simulink model "Mainframe"  (R2021a)
settings: Solver=FixedStepAuto  StartTime=0.0  StopTime=60  FixedStep=0.001  RelTol=1e-3
values from neighbouring files (symbols this model uses):
  den_lpf_d = den_lpf20    [Mainframe_init.m]    (also in load_autopilot.m)
  Emulated_FCC_IO_Delay = 7    [Mainframe_init.m]
  Enable_Gyros = 0    [Mainframe_init.m]
  Enable_INS = 0    [Mainframe_init.m]
  num_lpf_d = num_lpf20    [Mainframe_init.m]    (also in load_autopilot.m)
undefined symbols (not defined in the file or in its folder): act_dmp, act_omega, Actuator, Aerodynamics, aMode, Autopilot, AUX, c_b_WGS, c_be, c_flat, c_grav, c_h_geop0, c_h_geope, c_pa0, c_pe, c_r0, c_rot, c_rsma, c_Tmp0, d_siB_0, d_siB_max, d_siB_min, dd_siB_max, dd_siB_min, dev, DiscIntNeverNeededParam, e_pa, e_Tmp, fin_maxrate, flag_I_act_switch, flag_I_aero_switch, flag_I_flat, flag_I_gravity_switch, flag_I_rot, hcr, HIL_Data, JMMM_0, JMMM_e, JSPB_e, lat_0, lon_0, Mass_Props, mB_0, mM_0, mM_e, National_Instruments, Newton, pBII_0, PCIe, pMPB, pNPB, propellant_kg, prp_FBPB, prp_mdot, prp_T, pSPB, pwm_output1, qEG_0, qIB_0, qIE_0 ... (+31)
libraries: simulink_extras x38, simulink x31, custom_blocks x11, sldrtlib x10, aerolibcommonsys x4, px4Sensorslib x3, px4lib x3, aerolibnav x1
(part 2 of 17)

== system Mainframe/Non-linear Flight Dynamic Model/GRM_Airframe ==
  siB_cmd : Inport
  T_sim_glbl : Inport  Port=2
  Bus Creator : BusCreator  Inputs=9
  aerodynamics : Subsystem
  environment : Subsystem
  fin_actuators : Subsystem
  forces_moments : Subsystem
  gravity : Subsystem
  input : Subsystem
  motion_kinematics : Subsystem
  propulsion : Subsystem
  rb_eom : Subsystem
  stream_flow : Subsystem
  weight_and_balance : Subsystem
  airfr : Outport  VectorParamsAs1DForOutWhenUnconnected=off
  wires:
  forces_moments/1(for_mom_bus) -> rb_eom/2(for_mom)
  [env] -> Bus Creator/9
  [fin] -> Bus Creator/7
  [motion_kin] -> Bus Creator/6
  [env_glbl] -> aerodynamics/4(env_glbl)
  aerodynamics/1(aero) -> forces_moments/1(aero), [aero]
  [motion_kin] -> rb_eom/1(mot_kin)
  weight_and_balance/1(wab) -> rb_eom/3(wab), gravity/2(wab), [wab], propulsion/2(wab)
  [wab] -> aerodynamics/3(wab)
  [str_flow] -> Bus Creator/5
  [motion_kin] -> forces_moments/2(motion_kin)
  motion_kinematics/1(motion_kin) -> stream_flow/2(motion_kin), [motion_kin]
  [grav] -> Bus Creator/3
  Bus Creator/1 -> airfr/1  "airfr_bus"
  [aero] -> Bus Creator/4
  environment/1(env) -> [env], stream_flow/3(env), gravity/1(env)
  [prp] -> forces_moments/4(prp)
  [prp] -> Bus Creator/8
  stream_flow/1(str_flow) -> [str_flow], aerodynamics/1(str_flow)
  input/1(cmd_bus) -> fin_actuators/1(cmd)
  [wab] -> Bus Creator/2
  gravity/1(grav) -> [grav], forces_moments/3(grav)
  T_sim_glbl/1 -> [env_glbl], environment/2(env_glbl), weight_and_balance/1(env_glb), propulsion/1(env_glbl)
  siB_cmd/1 -> input/1(siB_cmd)
  rb_eom/1(flight_dyn) -> environment/1(flight_dyn), motion_kinematics/1(flight_dyn), stream_flow/1(flight_dyn), Bus Creator/1
  fin_actuators/1(fin) -> [fin], aerodynamics/2(fin)
  propulsion/1(prp) -> [prp]

== system Mainframe/Non-linear Flight Dynamic Model/Stop-Condition ==
  States : Inport
  AND : Logic  Inputs=3  IconShape=distinctive  AllPortsSameDT=off  OutDataTypeStr=boolean
  Bus Selector1 : BusSelector  OutputSignals=POS_NED.POS_z_NED_m,POS_NED_dot.POS_z_NED_dot_m
  Compare To Constant : Subsystem  mask(Compare To Constant){relop=>, const=-700, OutDataTypeStr=boolean, ZeroCross=on}
      mask prompts: relop "Simulink:masks:Operator_MP"; const "Simulink:masks:ConstantValue_MP"; OutDataTypeStr "Simulink:masks:OutputDataType_MP"; ZeroCross "Simulink:masks:EnableZerocrossingDetection_MP"
      mask help: Simulink:masks:CompareToConstant_MD
      mask init:
      | blkName = gcb;
      | 
      | if strcmp(get_param(gcbh,'OutDataTypeStr'),'boolean')
      | 	setValue = 'boolean';
      | else
      | 	setValue = 'fixdt(0, 8)';
      | end
      | 
      | set_param([blkName,'/Compare'],'relop',relop, ...
      | 	'OutDataTypeStr', setValue, 'ZeroCross', ZeroCross);
      | 
      | str = [relop,' C']; %default
      | 
      | const_str = get_param(blkName, 'const');
      | const_val = str2num(const_str);
      | 
      | if isempty(const_val) %#ok<ST2NM>
      |     %Expression/Variable
      |     str = [relop, ' ', strtrim(const_str)];
      | else
      |     if length(const_val) == 1 
      |         if Simulink.data.isSupportedEnumClass(class(const_val))
      |             % Special Handling for Enumerations
      |             if Simulink.data.getEnumTypeInfo(class(const_val), 'AddClassNameToEnumNames')
      |                 str = [relop, ' ', strtrim(const_str)];
      |             else
      |                 str = [relop, ' ', char(const_val)];
      |             end
      |         elseif(isfloat(const_val) || isinteger(const_val) || islogical(const_val)) 
      |                 str = [relop, ' ', num2str(const_val)];
      |         end
      |     end
      | end
      mask TypeOptions relop: == | ~= | < | <= | >= | >
      mask TypeOptions OutDataTypeStr: Simulink:masks:uint8 | Simulink:masks:boolean
      mask Callback ZeroCross: sl('zeroCrossEnable', gcbh);
      mask Display: disp(str)
  Compare To Constant1 : Subsystem  mask(Compare To Constant){relop=>, const=0, OutDataTypeStr=boolean, ZeroCross=on}
      mask prompts: relop "Simulink:masks:Operator_MP"; const "Simulink:masks:ConstantValue_MP"; OutDataTypeStr "Simulink:masks:OutputDataType_MP"; ZeroCross "Simulink:masks:EnableZerocrossingDetection_MP"
      mask help: Simulink:masks:CompareToConstant_MD
      mask init: same as Mainframe/Non-linear Flight Dynamic Model/Stop-Condition/Compare To Constant
      mask TypeOptions relop: == | ~= | < | <= | >= | >
      mask TypeOptions OutDataTypeStr: Simulink:masks:uint8 | Simulink:masks:boolean
      mask Callback ZeroCross: sl('zeroCrossEnable', gcbh);
      mask Display: disp(str)
  From4 : From  Commented=on  GotoTag=HIL_Ready  TagVisibility=global
  Stop Simulation : Stop
  wires:
  Bus Selector1/1 -> Compare To Constant/1(u)  "<POS_z_NED_m>"
  States/1 -> Bus Selector1/1
  Compare To Constant/1(y) -> AND/2
  AND/1 -> Stop Simulation/1
  From4/1 -> AND/1
  Bus Selector1/2 -> Compare To Constant1/1(u)  "<POS_z_NED_dot_m>"
  Compare To Constant1/1(y) -> AND/3

== system Mainframe/Non-linear Flight Dynamic Model/Subsystem1 ==
  Control Surface Deflections : Inport
  Envoronment : Inport  Port=2
  Enable : EnablePort
  Extract States : Subsystem
  Fin Deflections : Subsystem
  GRM_Airframe : Subsystem
      mask Display: image('$imagefile'); % Use "Edit Image" on toolstrip to change.
  Missile States : Outport
  wires:
  GRM_Airframe/1(airfr) -> Extract States/1(airfr_bus)
  Control Surface Deflections/1 -> Fin Deflections/1(Servo Deflections)
  Envoronment/1 -> GRM_Airframe/2(T_sim_glbl)
  Extract States/1(States) -> Missile States/1
  Fin Deflections/1(afinB) -> GRM_Airframe/1(siB_cmd)

== system Mainframe/Non-linear Flight Dynamic Model/Translate Fins ==
  Servo Deflections : Inport
  Add : Sum
  Bus Selector : BusSelector  OutputSignals=Fin_1,Fin_2,Fin_3,Fin_4
  Constant1 : Constant  Value=unc_fin_def_roll
  Constant2 : Constant  Value=unc_fin_def_pitch
  Constant3 : Constant  Value=unc_fin_def_yaw
  Degrees to Radians : Subsystem  mask(DegreesToRadians){}
      mask help: SimulinkBlocks:simulink_extras:DegreesToRadians_MD
      mask Help: web([docroot '/simulink/ref_extras/degreestoradians.html'])
      mask Display: disp('D2R')
  Degrees to Radians1 : Subsystem  mask(DegreesToRadians){}
      mask help: SimulinkBlocks:simulink_extras:DegreesToRadians_MD
      mask Help: web([docroot '/simulink/ref_extras/degreestoradians.html'])
      mask Display: disp('D2R')
  Degrees to Radians2 : Subsystem  mask(DegreesToRadians){}
      mask help: SimulinkBlocks:simulink_extras:DegreesToRadians_MD
      mask Help: web([docroot '/simulink/ref_extras/degreestoradians.html'])
      mask Display: disp('D2R')
  Vector Concatenate : Concatenate  NumInputs=4
  Vector Concatenate1 : Concatenate  NumInputs=3
  control_allocation : Subsystem
  afinB : Outport
  wires:
  Degrees to Radians2/1(Radians out) -> Vector Concatenate1/3
  Vector Concatenate1/1 -> control_allocation/1(fin_cmd)  "fin_cmd"
  Constant1/1 -> Degrees to Radians/1(Degrees in)  "xi_cmd"
  Degrees to Radians1/1(Radians out) -> Vector Concatenate1/2
  Degrees to Radians/1(Radians out) -> Vector Concatenate1/1
  Constant3/1 -> Degrees to Radians2/1(Degrees in)  "ze_cmd"
  Constant2/1 -> Degrees to Radians1/1(Degrees in)  "et_cmd"
  Bus Selector/2 -> Vector Concatenate/2  "<Fin_2>"
  Servo Deflections/1 -> Bus Selector/1
  Bus Selector/1 -> Vector Concatenate/1  "<Fin_1>"
  Bus Selector/4 -> Vector Concatenate/4  "<Fin_4>"
  Vector Concatenate/1 -> Add/1
  Bus Selector/3 -> Vector Concatenate/3  "<Fin_3>"
  control_allocation/1(siB_cmd) -> Add/2
  Add/1 -> afinB/1  "siB_cmd"

== system Mainframe/Real FCC/Enabled Subsystem ==
  Hold : Inport
  Trigger : TriggerPort  VariantControl=Variant  PortDimensions=1
  Pass : Outport
  wires:
  Hold/1 -> Pass/1

== system Mainframe/Real Servos/Reset Encoders ==
  Reset Encoders : Inport
  Encoder Readings : Inport  Port=2
  NOT : Logic  Operator=NOT  IconShape=distinctive  AllPortsSameDT=off  OutDataTypeStr=boolean
  Sum : Sum  Inputs=-+|
  Triggered Subsystem : Subsystem  TreatAsAtomicUnit=on
  Fin Angles : Outport
  wires:
  Encoder Readings/1 -> Sum/2, Triggered Subsystem/1(In1)
  Triggered Subsystem/1(Out1) -> Sum/1
  Reset Encoders/1 -> NOT/1
  Sum/1 -> Fin Angles/1
  NOT/1 -> Triggered Subsystem/Enable

== system Mainframe/Servos/Emulated Servos ==
  FCC Data : Inport
  Bus Creator : BusCreator  Inputs=4
  Bus Selector : BusSelector  OutputSignals=Control Surface Cmd.Fin_1_Cmd_rad,Control Surface Cmd.Fin_2_Cmd_rad,Control Surface Cmd.Fin_3_Cmd_rad,Control Surface Cmd.Fin_4_Cmd_rad
  Transfer Fcn{1..4} (4 alike) : TransferFcn  Numerator=33770  Denominator=[1 395.7 33770]
  Fin Deflections : Outport
  wires:
  FCC Data/1 -> Bus Selector/1
  Bus Selector/1 -> Transfer Fcn1/1  "<Fin_1_Cmd_rad>"
  Bus Selector/2 -> Transfer Fcn2/1  "<Fin_2_Cmd_rad>"
  Bus Selector/3 -> Transfer Fcn3/1  "<Fin_3_Cmd_rad>"
  Bus Selector/4 -> Transfer Fcn4/1  "<Fin_4_Cmd_rad>"
  Bus Creator/1 -> Fin Deflections/1
  Transfer Fcn1/1 -> Bus Creator/1  "Fin_1"
  Transfer Fcn2/1 -> Bus Creator/2  "Fin_2"
  Transfer Fcn3/1 -> Bus Creator/3  "Fin_3"
  Transfer Fcn4/1 -> Bus Creator/4  "Fin_4"

== system Mainframe/Servos/Real Servos ==
  FCC Data : Inport
  Bus Creator : BusCreator  Inputs=4
  Demux : Demux
  Encoder Input : sldrtlib/Encoder Input  SampleTime=0.001  MaxMissedTicks=10  ShowMissedTicks=off  YieldWhenWaiting=off  DrvName=National_Instruments/PCIe-6321  DrvAddress=4294967295  DrvOptions=[0 0 0 2 2 2 2]  Channels=1:4  QuadMode=3  IndexPulse=1  InputFilter=Inf  DataType=1
      settings: AttributesFormatString=National Instruments\nPCIe-6321 [auto]
  Reset Encoders : Subsystem
  Terminator : Terminator
  Ticks to rads : Gain  Gain=2*pi/4096
  Fin Deflections : Outport
  wires:
  Encoder Input/1 -> Ticks to rads/1
  FCC Data/1 -> Terminator/1
  Bus Creator/1 -> Fin Deflections/1
  Demux/3 -> Bus Creator/3  "Fin_3"
  Demux/2 -> Bus Creator/2  "Fin_2"
  Demux/1 -> Bus Creator/1  "Fin_1"
  Demux/4 -> Bus Creator/4  "Fin_4"
  [HIL_Ready] -> Reset Encoders/1(Reset Encoders)
  Ticks to rads/1 -> Reset Encoders/2(Encoder Readings)
  Reset Encoders/1(Fin Angles) -> Demux/1

== system Mainframe/Virtual IMU/Gravity Vector ==
  Phi : Inport
  Theta : Inport  Port=2
  Cos : Trigonometry
  Cos1 : Trigonometry
  Cos2 : Trigonometry  Operator=cos
  Cos3 : Trigonometry  Operator=cos
  Multiply : Gain  Gain=9.81
  Multiply1 : Gain  Gain=9.81
  Multiply2 : Gain  Gain=-9.81
  Product : Product
  Product1 : Product
  Vector Concatenate1 : Concatenate  NumInputs=3
  g : Outport
  wires:
  Vector Concatenate1/1 -> g/1
  Cos/1 -> Multiply2/1
  Product/1 -> Multiply/1
  Cos1/1 -> Product/1
  Theta/1 -> Cos/1, Cos2/1
  Multiply/1 -> Vector Concatenate1/2
  Phi/1 -> Cos3/1, Cos1/1
  Product1/1 -> Multiply1/1
  Multiply1/1 -> Vector Concatenate1/3
  Multiply2/1 -> Vector Concatenate1/1
  Cos2/1 -> Product1/1, Product/2
  Cos3/1 -> Product1/2

== system Mainframe/Emulated FCC/Emulated Pixhawk/Autopilot ==
  Cmd : Inport
  IMU Data : Inport  Port=2
  INS Data : Inport  Port=3
  Bus Creator3 : BusCreator  Inputs=3
  Bus Selector : BusSelector  OutputSignals=phi_cmd
  Bus Selector1 : BusSelector  OutputSignals=gyro_x
  Bus Selector2 : BusSelector  OutputSignals=phi,z,p
  Calculate U : Subsystem
  Discrete Transfer Fcn : DiscreteTransferFcn  Numerator=[num_lpf_d]  Denominator=[den_lpf_d]
  Gain : Gain  Gain=-1
  Manual Switch : ManualSwitch
  Phi_Control : Subsystem
  Zero : Constant  Value=0  OutDataTypeStr=Inherit: Inherit via back propagation
  Attitude_Commands : Outport  VectorParamsAs1DForOutWhenUnconnected=off
  wires:
  Bus Selector1/1 -> Discrete Transfer Fcn/1  "<gyro_x>"
  IMU Data/1 -> Bus Selector1/1
  Calculate U/1(U) -> Phi_Control/5(V_mps)
  Zero/1 -> [Delta_Cmd_Psi], [Delta_Cmd_Theta]
  [Delta_Cmd_Phi] -> Bus Creator3/1  "Phi_Cmd_rad"
  [Delta_Cmd_Theta] -> Bus Creator3/2  "Theta_Cmd_rad"
  Bus Creator3/1 -> Attitude_Commands/1
  [Delta_Cmd_Psi] -> Bus Creator3/3  "Psi_Cmd_rad"
  Bus Selector/1 -> Phi_Control/1(phi_cmd_rad)  "<phi_cmd>"
  Cmd/1 -> Bus Selector/1
  INS Data/1 -> Calculate U/1(INS Data), Bus Selector2/1
  Bus Selector2/1 -> Phi_Control/2(phi_rad)  "<phi>"
  [rst] -> Phi_Control/4(Reset Integrators)
  Bus Selector2/2 -> Gain/1  "<z>"
  Gain/1 -> Phi_Control/6(h_m)
  Phi_Control/1(dela_cmd_rad) -> [Delta_Cmd_Phi]  "Phi_Cmd_rad"
  Discrete Transfer Fcn/1 -> Manual Switch/1
  Bus Selector2/3 -> Manual Switch/2  "<p>"
  Manual Switch/1 -> Phi_Control/3(p_rps)

== system Mainframe/Emulated FCC/Emulated Pixhawk/Convert to Bus ==
  Input : Inport  OutDataTypeStr=single
  100Hz Reset : Subsystem
  Bus Creator1 : BusCreator  Inputs=6
  Bus Creator2 : BusCreator  Inputs=12
  Bus Creator3 : BusCreator  Inputs=1
  Demux : Demux  Outputs=23
  Heartbeat : Outport  InitialOutput=0
  Ext. Commands : Outport  Port=2  OutDataTypeStr=single  InitialOutput=0
  Enable INS Flag : Outport  Port=3  InitialOutput=0
  Missile States : Outport  Port=4  OutDataTypeStr=single  InitialOutput=[0 0 0 0 0 0 0 0 0 0]
  Real Gyros Flag : Outport  Port=5  InitialOutput=0
  Virtual IMU Data : Outport  Port=6  OutDataTypeStr=single  InitialOutput=[0 0 0 0 0 0 0 0 0 0]
  tag scope: FCC_Enable=global, rst=global
  wires:
  Demux/22 -> Bus Creator2/12  "psi"
  Demux/21 -> Bus Creator2/11  "theta"
  Demux/20 -> Bus Creator2/10  "phi"
  Demux/4 -> Real Gyros Flag/1  "Real Gyros Flag"
  Demux/5 -> Bus Creator2/1  "u"
  Demux/18 -> Bus Creator1/5  "gyro_y"
  Bus Creator1/1 -> Virtual IMU Data/1
  Demux/16 -> Bus Creator1/3  "acc_z"
  Demux/9 -> Bus Creator2/5  "y"
  Demux/14 -> Bus Creator1/1  "acc_x"
  Demux/17 -> Bus Creator1/4  "gyro_x"
  Demux/15 -> Bus Creator1/2  "acc_y"
  Demux/19 -> Bus Creator1/6  "gyro_z"
  Demux/12 -> Bus Creator2/8  "q"
  Demux/7 -> Bus Creator2/3  "w"
  Demux/10 -> Bus Creator2/6  "z"
  Demux/6 -> Bus Creator2/2  "v"
  Demux/11 -> Bus Creator2/7  "p"
  Demux/13 -> Bus Creator2/9  "r"
  Demux/23 -> Bus Creator3/1  "phi_cmd"
  Demux/8 -> Bus Creator2/4  "x"
  Bus Creator3/1 -> Ext. Commands/1
  Bus Creator2/1 -> Missile States/1
  Demux/1 -> [FCC_Enable]  "EnableFCC"
  Input/1 -> Demux/1
  Demux/2 -> 100Hz Reset/1(Heartbeat), Heartbeat/1  "Hearbeat"
  Demux/3 -> Enable INS Flag/1  "Enable INS Flag"
  100Hz Reset/1(RST) -> [rst]

== system Mainframe/Emulated FCC/Emulated Pixhawk/Convert to Vector ==
  Fin Deflections : Inport
  Heartbeat : Inport  Port=2
  INS Data : Inport  Port=3
  Real Gyro Data : Inport  Port=4
  Debug Port : Inport  Port=5
  Bus Selector1 : BusSelector  OutputSignals=Fin_1_Cmd_rad,Fin_2_Cmd_rad,Fin_3_Cmd_rad,Fin_4_Cmd_rad
  Bus Selector2 : BusSelector  OutputSignals=gyro_x,gyro_y,gyro_z
  Bus Selector3 : BusSelector  OutputSignals=u,v,w,x,y,z,p,q,r
  Cast To Single : DataTypeConversion  OutDataTypeStr=single
  Vector Concatenate : Concatenate  NumInputs=18
  To HIL : Outport
  wires:
  Bus Selector1/3 -> Vector Concatenate/4  "<Fin_3_Cmd_rad>"
  Bus Selector1/4 -> Vector Concatenate/5  "<Fin_4_Cmd_rad>"
  Heartbeat/1 -> Vector Concatenate/1
  Bus Selector1/1 -> Vector Concatenate/2  "<Fin_1_Cmd_rad>"
  Bus Selector1/2 -> Vector Concatenate/3  "<Fin_2_Cmd_rad>"
  Vector Concatenate/1 -> Cast To Single/1
  Fin Deflections/1 -> Bus Selector1/1
  Cast To Single/1 -> To HIL/1
  Real Gyro Data/1 -> Bus Selector2/1
  Bus Selector3/7 -> Vector Concatenate/15  "<p>"
  Bus Selector3/5 -> Vector Concatenate/13  "<y>"
  Bus Selector3/4 -> Vector Concatenate/12  "<x>"
  Bus Selector3/9 -> Vector Concatenate/17  "<r>"
  Bus Selector3/3 -> Vector Concatenate/11  "<w>"
  Bus Selector2/3 -> Vector Concatenate/8  "<gyro_z>"
  Debug Port/1 -> Vector Concatenate/18
  Bus Selector3/1 -> Vector Concatenate/9  "<u>"
  Bus Selector2/2 -> Vector Concatenate/7  "<gyro_y>"
  Bus Selector2/1 -> Vector Concatenate/6  "<gyro_x>"
  Bus Selector3/8 -> Vector Concatenate/16  "<q>"
  INS Data/1 -> Bus Selector3/1
  Bus Selector3/6 -> Vector Concatenate/14  "<z>"
  Bus Selector3/2 -> Vector Concatenate/10  "<v>"

== system Mainframe/Emulated FCC/Emulated Pixhawk/Fin Allocation ==
  Attitude Cmd : Inport
  Bus Creator : BusCreator  Inputs=4
  Bus Selector : BusSelector  OutputSignals=Phi_Cmd_rad,Theta_Cmd_rad,Psi_Cmd_rad
  Demux : Demux
  Vector Concatenate1 : Concatenate  NumInputs=3
  control_allocation : Subsystem
  Fin Cmd : Outport  VectorParamsAs1DForOutWhenUnconnected=off
  wires:
  Demux/4 -> Bus Creator/4  "Fin_4_Cmd_rad"
  control_allocation/1(siB_cmd) -> Demux/1
  Bus Selector/3 -> Vector Concatenate1/3  "<Psi_Cmd_rad>"
  Vector Concatenate1/1 -> control_allocation/1(fin_cmd)  "fin_cmd"
  Bus Selector/1 -> Vector Concatenate1/1  "<Phi_Cmd_rad>"
  Demux/3 -> Bus Creator/3  "Fin_3_Cmd_rad"
  Bus Selector/2 -> Vector Concatenate1/2  "<Theta_Cmd_rad>"
  Demux/1 -> Bus Creator/1  "Fin_1_Cmd_rad"
  Bus Creator/1 -> Fin Cmd/1
  Attitude Cmd/1 -> Bus Selector/1
  Demux/2 -> Bus Creator/2  "Fin_2_Cmd_rad"

== system Mainframe/Emulated FCC/Emulated Pixhawk/Gyro ==
  Bus Creator2 : BusCreator  Inputs=3
  Gyroscope : px4Sensorslib/Gyroscope  uorbTimeStamp=off  BlockingMode=off  BlockTimeout=1e-3  sampleTime=-1
      settings: SourceProductBaseCode=PX4AUTOPILOTS
  Terminator3 : Terminator
  Real Gyro Data : Outport
  wires:
  Gyroscope/1 -> Terminator3/1
  Bus Creator2/1 -> Real Gyro Data/1  "gyro"
  Gyroscope/4 -> Bus Creator2/3  "gyro_z"
  Gyroscope/2 -> Bus Creator2/1  "gyro_x"
  Gyroscope/3 -> Bus Creator2/2  "gyro_y"

== system Mainframe/Emulated FCC/Emulated Pixhawk/IMU - Merge ==
  Real Gyro Flag : Inport
  HIL IMU : Inport  Port=2
  Real Gyro : Inport  Port=3
  Bus Creator1 : BusCreator  Inputs=6
  Bus Creator2 : BusCreator  Inputs=6
  Bus Selector : BusSelector  OutputSignals=acc_x,acc_y,acc_z
  Bus Selector1 : BusSelector  OutputSignals=gyro_x,gyro_y,gyro_z
  Bus Selector2 : BusSelector  OutputSignals=acc_x,acc_y,acc_z,gyro_x,gyro_y,gyro_z
  Switch : Switch  Criteria=u2 > Threshold
  IMU Data : Outport
  wires:
  Real Gyro Flag/1 -> Switch/2
  Real Gyro/1 -> Bus Selector1/1
  HIL IMU/1 -> Bus Selector2/1, Bus Selector/1
  Bus Selector/3 -> Bus Creator1/3  "<acc_z>"
  Bus Selector/1 -> Bus Creator1/1  "<acc_x>"
  Bus Selector/2 -> Bus Creator1/2  "<acc_y>"
  Bus Selector1/1 -> Bus Creator1/4  "<gyro_x>"
  Bus Selector1/3 -> Bus Creator1/6  "<gyro_z>"
  Bus Creator1/1 -> Switch/1
  Bus Selector1/2 -> Bus Creator1/5  "<gyro_y>"
  Bus Selector2/5 -> Bus Creator2/5  "<gyro_y>"
  Bus Selector2/6 -> Bus Creator2/6  "<gyro_z>"
  Bus Selector2/4 -> Bus Creator2/4  "<gyro_x>"
  Bus Selector2/2 -> Bus Creator2/2  "<acc_y>"
  Bus Selector2/1 -> Bus Creator2/1  "<acc_x>"
  Bus Selector2/3 -> Bus Creator2/3  "<acc_z>"
  Bus Creator2/1 -> Switch/3
  Switch/1 -> IMU Data/1

== system Mainframe/Emulated FCC/Emulated Pixhawk/Inertial Navigation System ==
  Enable INS Flag : Inport
  Missile States : Inport  Port=2
  IMU Data : Inport  Port=3
  INS (INCOMPLETE) : Subsystem
  Switch : Switch  Criteria=u2 > Threshold
  INS Data : Outport
  wires:
  Enable INS Flag/1 -> Switch/2
  IMU Data/1 -> INS (INCOMPLETE)/1(IMU Data)
  Switch/1 -> INS Data/1
  Missile States/1 -> Switch/3
  INS (INCOMPLETE)/1(INS Data) -> Switch/1

== system Mainframe/Emulated FCC/Emulated Pixhawk/Servo Commands ==
  Fin Cmd : Inport
  100Hz Progress : Subsystem
  AND : Logic  IconShape=distinctive  AllPortsSameDT=off  OutDataTypeStr=boolean
  Add{,1..3} (4 alike) : Sum
  Bus Selector : BusSelector  OutputSignals=Fin_1_Cmd_rad,Fin_2_Cmd_rad,Fin_3_Cmd_rad,Fin_4_Cmd_rad
  Cast To Boolean : DataTypeConversion  OutDataTypeStr=boolean
  Cast To Double{,1..3} (4 alike) : DataTypeConversion  OutDataTypeStr=uint16
  Gain{,1..3} (4 alike) : Gain  Gain=1000/91
  One{,1..3} (4 alike) : Constant  Value=1500  OutDataTypeStr=Inherit: Inherit via back propagation
  One4 : Constant  Value=0  OutDataTypeStr=boolean
  PX4 PWM Output1 : px4lib/PX4 PWM Output  pwmDevice=AUX (/dev/pwm_output1)  pwmChannel1_=on  pwmChannel2_=on  pwmChannel3_=on  pwmChannel4_=on  pwmChannel5_=off  pwmChannel6_=off  pwmChannel7_=off  pwmChannel8_=off  forceTerminateFailsafe=off  outputErrorStatus=off
      settings: SourceProductBaseCode=PX4AUTOPILOTS
  Radians to Degrees{,1..3} (4 alike) : simulink_extras/Transformations/Radians to Degrees
  Saturation{,1..3} (4 alike) : Saturate  UpperLimit=20  LowerLimit=-20
  wires:
  Saturation2/1 -> Gain2/1
  Cast To Double3/1 -> PX4 PWM Output1/6
  One4/1 -> PX4 PWM Output1/2
  One/1 -> Add/2
  One2/1 -> Add2/2
  Add1/1 -> Cast To Double1/1
  Gain2/1 -> Add2/1
  AND/1 -> Cast To Boolean/1
  Radians to Degrees1/1 -> Saturation1/1
  Cast To Double2/1 -> PX4 PWM Output1/5
  Add2/1 -> Cast To Double2/1
  Fin Cmd/1 -> Bus Selector/1
  Cast To Double1/1 -> PX4 PWM Output1/4
  Bus Selector/2 -> Radians to Degrees1/1  "<Fin_2_Cmd_rad>"
  Gain/1 -> Add/1
  Bus Selector/4 -> Radians to Degrees3/1  "<Fin_4_Cmd_rad>"
  One3/1 -> Add3/2
  Saturation/1 -> Gain/1
  Gain1/1 -> Add1/1
  Saturation3/1 -> Gain3/1
  Gain3/1 -> Add3/1
  Radians to Degrees3/1 -> Saturation3/1
  Bus Selector/1 -> Radians to Degrees/1  "<Fin_1_Cmd_rad>"
  Bus Selector/3 -> Radians to Degrees2/1  "<Fin_3_Cmd_rad>"
  Saturation1/1 -> Gain1/1
  Cast To Double/1 -> PX4 PWM Output1/3
  Add3/1 -> Cast To Double3/1
  Radians to Degrees2/1 -> Saturation2/1
  [FCC_Enable] -> AND/1
  Radians to Degrees/1 -> Saturation/1
  100Hz Progress/1(RST) -> AND/2
  One1/1 -> Add1/2
  Add/1 -> Cast To Double/1
  Cast To Boolean/1 -> PX4 PWM Output1/1

== system Mainframe/Flight Control Computer/FCC - Real or Emulated/Emulated FCC ==
  Input Data : Inport
  100 Hz : DiscretePulseGenerator  Commented=on  PulseType=Time based  Period=0.01  PulseWidth=50
  Delay : Delay  DelayLength=Emulated_FCC_IO_Delay  SampleTime=0.001
  Delay1 : Delay  DelayLength=Emulated_FCC_IO_Delay  SampleTime=0.001
  Emulated Pixhawk : Subsystem  Commented=on
  PixBlock2 : Subsystem
  Output Data : Outport
  wires:
  100 Hz/1 -> Emulated Pixhawk/Trigger
  Input Data/1 -> Delay/1
  Delay/1 -> PixBlock2/1(Serial In)
  PixBlock2/1(Serial Out) -> Delay1/1
  Delay1/1 -> Output Data/1

== system Mainframe/Flight Control Computer/FCC - Real or Emulated/Real FCC ==
  Input Data : Inport
  Enabled Subsystem : Subsystem  TreatAsAtomicUnit=on
  Extract Message : MATLAB Function  TreatAsAtomicUnit=on
  Packet Input : sldrtlib/Packet Input  SampleTime=0.001  MaxMissedTicks=10  ShowMissedTicks=off  YieldWhenWaiting=on  DrvName=Standard_Devices/Serial_Port  DrvAddress=3  DrvOptions=[115200 8 0 0 0 0 0 0]  PacketSize=FCC_message_size  DataTypes=FCC_types  ShowReady=on  ShowError=off  PacketID=1  ByteOrder=1  ShowTimestamp=off
      settings: AttributesFormatString=Serial Port [3]
  Packet Output : sldrtlib/Packet Output  SampleTime=0.01  MaxMissedTicks=10  ShowMissedTicks=off  YieldWhenWaiting=on  DrvName=Standard_Devices/Serial_Port  DrvAddress=3  DrvOptions=[115200 8 0 0 0 0 0 0]  PacketSize=23*4  DataTypes='23*single'  ShowReady=off  ShowError=off  PacketID=1  ByteOrder=1  InitialValue=[]  FinalValue=[]
      settings: AttributesFormatString=Serial Port [3]
  Terminator1 : Terminator
  Output Data : Outport
  wires:
  Input Data/1 -> Packet Output/1
  Packet Input/1 -> Enabled Subsystem/1(Hold)
  Enabled Subsystem/1(Pass) -> Extract Message/1(packet)
  Packet Input/2 -> Enabled Subsystem/Trigger
  Extract Message/2(Extracted_Data) -> Output Data/1
  Extract Message/1(Error_Msg) -> Terminator1/1

== system Mainframe/Flight Control Computer/Heartbeat Check/In Sync ==
  note: This block ensures the Pixhawk is connected and functioning correctly
  send : Inport
  receive : Inport  Port=2
  Cast To Single : DataTypeConversion  OutDataTypeStr=single
  Mux : Mux  Inputs=2
  Rate Transition : RateTransition  OutPortSampleTime=0.001
  Rate Transition1 : RateTransition  OutPortSampleTime=0.001
  Heartbeat Sync : Outport
  wires:
  receive/1 -> Rate Transition1/1  "receive"
  send/1 -> Rate Transition/1
  Rate Transition/1 -> Mux/1
  Rate Transition1/1 -> Cast To Single/1
  Mux/1 -> Heartbeat Sync/1
  Cast To Single/1 -> Mux/2

== system Mainframe/Flight Control Computer/Send to FCC/Heartbeat Counter ==
  note: Starting the heartbeat at negative values prevents unwanted FCC behaviour on startup
  Cast To Double14 : DataTypeConversion  OutDataTypeStr=single
  Heartbeat : simulink/Sources/Counter Free-Running  NumBits=16  tsamp=-1
  Subtract : Sum  Inputs=+-
  Zero : Constant  Value=1000  OutDataTypeStr=Inherit: Inherit via back propagation
  Out1 : Outport
  wires:
  Heartbeat/1 -> Cast To Double14/1
  Zero/1 -> Subtract/2
  Cast To Double14/1 -> Subtract/1  "send"
  Subtract/1 -> Out1/1

== system Mainframe/Flight Gear Simulator/Flight Simulator On/Flat Earth to LLA ==
  Xe : Inport  Unit=m
  ground height : Inport  Port=2  Unit=m
  Disallow CGS : UnitConfiguration  UnitSystemsStr=English,SI,SI (extended)  AllowAllUnitSystems=off
  LatLong wrap : Subsystem
      mask init:
      | aeroicon('aeroblk')
      mask Display:
      | port_label('input',1,'[\mu l]','texmode','on')
      | port_label('output',1,'[\mu l]_{wrap}','texmode','on')
  LatLong wrap1 : Subsystem
      mask init:
      | aeroicon('aeroblk')
      mask Display:
      | port_label('input',1,'[\mu l]','texmode','on')
      | port_label('output',1,'[\mu l]_{wrap}','texmode','on')
  LongLat_offset : Subsystem
  Sel1 : Selector  InputPortWidth=3  IndexOptions=Index vector (dialog)  Indices=[1,2]  OutputSizes=1
  Sel2 : Selector  InputPortWidth=3  IndexOptions=Index vector (dialog)  Indices=3  OutputSizes=1
  Sum : Sum  Inputs=|++
  Sum1 : Sum  Inputs=-+
  "Xe " : InportShadow  Unit=m
  Ze2height : UnaryMinus
  initial_latg : Selector  InputPortWidth=2  IndexOptions=Index vector (dialog)  Indices=[1]  OutputSizes=1
  initial_pos : Constant  Value=LL0
  pos_deg : Subsystem
  mu l : Outport  Unit=deg  VectorParamsAs1DForOutWhenUnconnected=off
  h : Outport  Port=2  Unit=m  VectorParamsAs1DForOutWhenUnconnected=off
  wires:
  pos_deg/1(out) -> Sum/1
  LongLat_offset/1(DeltaLL_rad) -> pos_deg/1(in)
  LatLong wrap1/1(Lat/Long wrapped) -> initial_latg/1, Sum/2
  initial_pos/1 -> LatLong wrap1/1(LatLong)
  LatLong wrap/1(Lat/Long wrapped) -> mu l/1
  initial_latg/1 -> LongLat_offset/2(mu)
  "Xe "/1 -> Sel2/1
  Sel1/1 -> LongLat_offset/1(XY)
  ground height/1 -> Sum1/1
  Sum1/1 -> h/1
  Ze2height/1 -> Sum1/2  "alt"
  Sel2/1 -> Ze2height/1
  Sum/1 -> LatLong wrap/1(LatLong)
  Xe/1 -> Sel1/1

== system Mainframe/Flight Gear Simulator/Flight Simulator On/FlightGear Preconfigured 6DoF Animation ==
  In1 : Inport
  Angle Conversion : Subsystem
  Angle Conversion1 : Subsystem
  Demux : Demux  Outputs=6
  Pack net_fdm Packet for FlightGear : S-Function  FunctionName=saerofgpacknetfdm  Parameters=packetVersion, 'on','off','off','off','off','off', SampleTime  SFunctionDeploymentMode=off  EnableBusSupport=off
  PacketSize : Constant  Value=408
  Rate Transition : RateTransition  Integrity=off  Deterministic=off  OutPortSampleTime=SampleTime
  Simulation Pace : S-Function  FunctionName=saeroclockpacer  Parameters=SimulationPace,SleepMode,OutputPaceError,SampleTime  SFunctionDeploymentMode=off  EnableBusSupport=off  mask(Simulation Pace){SimulationPace=1, SleepMode=MATLAB Thread, OutputPaceError=off, SampleTime=SampleTime}
      mask prompts: SimulationPace "aeroblks:aeroblkanimutils:blockSimulationPaceParamSimulationpacesimsecperclocksec"; SleepMode "aeroblks:aeroblkanimutils:blockSimulationPaceParamSleepmode"; OutputPaceError "aeroblks:aeroblkanimutils:blockSimulationPaceParamOutputpaceerrorsec"; SampleTime "aeroblks:aeroblkanimutils:blockSimulationPaceParamSampletime1forinherited"
      mask help: aeroblks:aeroblkanimutils:blockSimulationPaceDesc
      mask init:
      | aeroicon('aeroblkpacer');
      settings: AttributesFormatString=%<SimulationPace> sec/sec
      mask Help: eval('asbhelp');
      mask TypeOptions SleepMode: aeroblks:aeroblkanimutils:blockSimulationPaceParamComboOff | aeroblks:aeroblkanimutils:blockSimulationPaceParamComboMATLABThread | aeroblks:aeroblkanimutils:blockSimulationPaceParamComboBusyWait | aeroblks:aeroblkanimutils:blockSimulationPaceParamComboAuto
      mask DialogControl SimulationPace Prompt: Simulation pace (sim sec per clock sec):
      mask DialogControl SleepMode Prompt: Sleep mode:
      mask DialogControl OutputPaceError Prompt: Output pace error (sec)
      mask DialogControl SampleTime Prompt: Sample time (-1 for inherited):
      mask Display:
      | text(0.5,0.60,'Set','horizontalAlignment','center');
      | text(0.5,0.40,'Pace','horizontalAlignment','center');
  UDP Send : S-Function  FunctionName=saerofgsend  Parameters=DestinationIpAddress,DestinationPort,-1,SampleTime,0  SFunctionDeploymentMode=off  EnableBusSupport=off
  Unit Sys : UnitConfiguration  UnitSystemsStr=SI,SI (extended)  AllowAllUnitSystems=off
  toSingle1 : DataTypeConversion  OutDataTypeStr=single
  toSingle2 : DataTypeConversion  OutDataTypeStr=single
  toSingle3 : DataTypeConversion  OutDataTypeStr=single
  wires:
  Angle Conversion1/1(out) -> Pack net_fdm Packet for FlightGear/2
  Angle Conversion/1(out) -> Pack net_fdm Packet for FlightGear/1
  Rate Transition/1 -> Demux/1
  toSingle3/1 -> Pack net_fdm Packet for FlightGear/6
  toSingle2/1 -> Pack net_fdm Packet for FlightGear/5
  toSingle1/1 -> Pack net_fdm Packet for FlightGear/4
  Pack net_fdm Packet for FlightGear/1 -> UDP Send/1
  In1/1 -> Rate Transition/1
  Demux/1 -> Angle Conversion/1(in)
  Demux/2 -> Angle Conversion1/1(in)
  Demux/3 -> Pack net_fdm Packet for FlightGear/3
  Demux/4 -> toSingle1/1
  Demux/5 -> toSingle2/1
  Demux/6 -> toSingle3/1
  PacketSize/1 -> UDP Send/2

== system Mainframe/Flight Gear Simulator/Flight Simulator On/FlightGear1 ==

== system Mainframe/Flight Simulator On/Flat Earth to LLA/LatLong wrap ==
  LatLong : Inport
  Constant : Constant  Value=180
  Constant1 : Constant  Value=0
  Demux : Demux  Outputs=2
  Latitude Wrap 90 : Subsystem  mask(LatitudeWrap90){}
      mask init:
      | aeroicon('aeroblk')
  Mux : Mux  Inputs=2
  Sum : Sum  Inputs=|++
  Switch1 : Switch  Criteria=u2 ~= 0
  Wrap Longitude : Subsystem
      mask init:
      | aeroicon('aeroblk');
  Lat/Long wrapped : Outport  VectorParamsAs1DForOutWhenUnconnected=off
  wires:
  Latitude Wrap 90/1(Lat wrapped) -> Mux/1
  Latitude Wrap 90/2(Wrap flag) -> Switch1/2
  Demux/1 -> Latitude Wrap 90/1(Lat)
  Wrap Longitude/1(Angle 180) -> Mux/2
  Mux/1 -> Lat/Long wrapped/1
  Sum/1 -> Wrap Longitude/1(Angle)
  Demux/2 -> Sum/2
  Switch1/1 -> Sum/1
  Constant1/1 -> Switch1/3
  Constant/1 -> Switch1/1
  LatLong/1 -> Demux/1

== system Mainframe/Flight Simulator On/Flat Earth to LLA/LatLong wrap1 ==
  LatLong : Inport
  Constant : Constant  Value=180
  Constant1 : Constant  Value=0
  Demux : Demux  Outputs=2
  Latitude Wrap 90 : Subsystem  mask(LatitudeWrap90){}
      mask init:
      | aeroicon('aeroblk')
  Mux : Mux  Inputs=2
  Sum : Sum  Inputs=|++
  Switch1 : Switch  Criteria=u2 ~= 0
  Wrap Longitude : Subsystem
      mask init:
      | aeroicon('aeroblk');
  Lat/Long wrapped : Outport  VectorParamsAs1DForOutWhenUnconnected=off
  wires:
  Latitude Wrap 90/1(Lat wrapped) -> Mux/1
  Latitude Wrap 90/2(Wrap flag) -> Switch1/2
  Demux/1 -> Latitude Wrap 90/1(Lat)
  Wrap Longitude/1(Angle 180) -> Mux/2
  Mux/1 -> Lat/Long wrapped/1
  Sum/1 -> Wrap Longitude/1(Angle)
  Demux/2 -> Sum/2
  Switch1/1 -> Sum/1
  Constant1/1 -> Switch1/3
  Constant/1 -> Switch1/1
  LatLong/1 -> Demux/1

== system Mainframe/Flight Simulator On/Flat Earth to LLA/LongLat_offset ==
  XY : Inport
  mu : Inport  Port=2
  Angle Conversion2 : Subsystem
  Demux : Demux  Outputs=2
  Find Radian/Distance : Subsystem
  Mux : Mux  Inputs=2
  SinCos : Trigonometry  Operator=sincos
  Sum : Sum  Inputs=|+-
  Sum1 : Sum  Inputs=|++
  rad lat : Product  RndMeth=Zero
  "rad long " : Product  RndMeth=Zero
  ref_pos : Constant  Value=psi
  x*cos : Product  RndMeth=Zero
  x*sin : Product  RndMeth=Zero
  y*cos : Product  RndMeth=Zero
  y*sin : Product  RndMeth=Zero
  DeltaLL_rad : Outport  VectorParamsAs1DForOutWhenUnconnected=off
  wires:
  mu/1 -> Find Radian/Distance/1(mu)
  Find Radian/Distance/1(dNorth) -> rad lat/2
  Find Radian/Distance/2(dEast) -> "rad long "/1
  rad lat/1 -> Mux/1
  "rad long "/1 -> Mux/2
  Mux/1 -> DeltaLL_rad/1
  Angle Conversion2/1(out) -> SinCos/1
  Demux/2 -> y*cos/1, y*sin/1
  Sum1/1 -> "rad long "/2
  y*cos/1 -> Sum1/2
  x*sin/1 -> Sum1/1
  Sum/1 -> rad lat/1
  y*sin/1 -> Sum/2
  SinCos/1 -> x*sin/2, y*sin/2
  x*cos/1 -> Sum/1
  SinCos/2 -> y*cos/2, x*cos/2
  Demux/1 -> x*sin/1, x*cos/1
  XY/1 -> Demux/1
  ref_pos/1 -> Angle Conversion2/1(in)

== system Mainframe/Flight Simulator On/Flat Earth to LLA/pos_deg ==
  in : Inport  Unit=rad
  Unit Conversion : UnitConversion
  out : Outport  Unit=deg  VectorParamsAs1DForOutWhenUnconnected=off
  wires:
  in/1 -> Unit Conversion/1
  Unit Conversion/1 -> out/1

== system Mainframe/Flight Simulator On/FlightGear Preconfigured 6DoF Animation/Angle Conversion ==
  in : Inport  Unit=deg
  Unit Conversion : UnitConversion
  out : Outport  Unit=rad  VectorParamsAs1DForOutWhenUnconnected=off
  wires:
  in/1 -> Unit Conversion/1
  Unit Conversion/1 -> out/1

== system Mainframe/Flight Simulator On/FlightGear Preconfigured 6DoF Animation/Angle Conversion1 ==
  in : Inport  Unit=deg
  Unit Conversion : UnitConversion
  out : Outport  Unit=rad  VectorParamsAs1DForOutWhenUnconnected=off
  wires:
  Unit Conversion/1 -> out/1
  in/1 -> Unit Conversion/1

== system Mainframe/Flight Table/Flight Table On/Configure Gimbals ==
  note: Set angles here
  note: Digital Output for "Enable Gimbal"
      | Analog Output for DC motors
      |
      | Digital Input for z-indexes
      | Encoder Input for encoders
  Analog Output : sldrtlib/Analog Output  SampleTime=0.001  MaxMissedTicks=10  ShowMissedTicks=off  YieldWhenWaiting=off  DrvName=National_Instruments/PCIe-6353  DrvAddress=4294967295  DrvOptions=[0 15 0 2 2 2 0]  Channels=1:3  RangeMode=1  VoltRange=1  InitialValue=[0 0 0]  FinalValue=[0 0 0]
      settings: AttributesFormatString=National Instruments\nPCIe-6353 [auto]
  Digital Input : sldrtlib/Digital Input  SampleTime=0.001  MaxMissedTicks=10  ShowMissedTicks=off  YieldWhenWaiting=off  DrvName=National_Instruments/PCIe-6353  DrvAddress=4294967295  DrvOptions=[0 15 0 2 2 2 0]  Channels=45:47  BitMode=1  DataType=1
      settings: AttributesFormatString=National Instruments\nPCIe-6353 [auto]  SourceProductBaseCode=WT
  Digital Output : sldrtlib/Digital Output  SampleTime=0.001  MaxMissedTicks=10  ShowMissedTicks=off  YieldWhenWaiting=off  DrvName=National_Instruments/PCIe-6353  DrvAddress=4294967295  DrvOptions=[0 15 0 2 2 2 0]  Channels=1:2  BitMode=1  InitialValue=[0 0]  FinalValue=[0 0]
      settings: AttributesFormatString=National Instruments\nPCIe-6353 [auto]  SourceProductBaseCode=WT
  Display : Display
  Enable gimbal : custom_blocks/Enable gimbal  yawOffset=0  pitchOffset=0  rollOffset=180-37
  Encoder Input : sldrtlib/Encoder Input  SampleTime=0.001  MaxMissedTicks=10  ShowMissedTicks=off  YieldWhenWaiting=off  DrvName=National_Instruments/PCIe-6353  DrvAddress=4294967295  DrvOptions=[0 15 0 2 2 2 0]  Channels=1:3  QuadMode=3  IndexPulse=1  InputFilter=Inf  DataType=1
      settings: AttributesFormatString=National Instruments\nPCIe-6353 [auto]
  Gimbal Motors : custom_blocks/Gimbal Motors
  Multiport Switch : MultiPortSwitch
  Subsystem : Subsystem
  Ticks To Degrees : Subsystem
  tag scope: GimbalDigitalInput=global, GimbalRawOutput=global
  wires:
  Gimbal Motors/1 -> Analog Output/1
  Digital Input/1 -> [GimbalDigitalInput]
  Enable gimbal/1 -> Digital Output/1
  Encoder Input/1 -> Ticks To Degrees/1(In1)
  Ticks To Degrees/1(Out1) -> [GimbalRawOutput]
  [Voltage1] -> Multiport Switch/2
  Multiport Switch/1 -> Gimbal Motors/1
  [Voltage2] -> Multiport Switch/3
  Subsystem/1(Stage) -> Display/1, Multiport Switch/1
  [Voltage3] -> Multiport Switch/4

== system Mainframe/Flight Table/Flight Table On/Current Attitude ==
  Bus Selector : BusSelector  OutputSignals=inertialYaw,inertialPitch,inertialRoll
  Convert To Inertial : custom_blocks/Convert To Inertial
  Degrees to Radians : simulink_extras/Transformations/Degrees to Radians
  Degrees to Radians1 : simulink_extras/Transformations/Degrees to Radians
  Degrees to Radians2 : simulink_extras/Transformations/Degrees to Radians
  gimbalPhi : Outport
  gimbalTheta : Outport  Port=2
  gimbalPsi : Outport  Port=3
  wires:
  Bus Selector/2 -> Degrees to Radians1/1  "<inertialPitch>"
  Bus Selector/3 -> Degrees to Radians2/1  "<inertialRoll>"
  Bus Selector/1 -> Degrees to Radians/1  "<inertialYaw>"
  Degrees to Radians2/1 -> gimbalPhi/1  "gimbalPhi"
  Degrees to Radians/1 -> gimbalPsi/1  "gimbalPsi"
  Degrees to Radians1/1 -> gimbalTheta/1  "gimbalTheta"
  [GimbalRawOutput] -> Convert To Inertial/1
  [offsets] -> Convert To Inertial/2
  Convert To Inertial/1 -> Bus Selector/1

== system Mainframe/Flight Table/Flight Table On/Stage 1 - Spin 360deg to find indexes ==
  Bus Creator : BusCreator  Inputs=3
  Constant : Constant  Value=400
  Constant1 : Constant  Value=400
  Constant2 : Constant  Value=400
  Gimbal Control : custom_blocks/Gimbal Input
  Index Locations : custom_blocks/Index Locations
  tag scope: Voltage1=global, offsets=global, stage1complete=global
  wires:
  Constant/1 -> Gimbal Control/1
  Index Locations/2 -> Bus Creator/2  "pitchAbsOffset"
  Constant2/1 -> Gimbal Control/3
  Index Locations/3 -> Bus Creator/3  "rollAbsOffset"
  Index Locations/1 -> Bus Creator/1  "yawAbsOffset"
  Constant1/1 -> Gimbal Control/2
  Index Locations/4 -> [stage1complete]
  Gimbal Control/1 -> [Voltage1]
  Bus Creator/1 -> [offsets]
  [GimbalDigitalInput] -> Index Locations/1
  [GimbalRawOutput] -> Gimbal Control/4, Index Locations/2

== system Mainframe/Flight Table/Flight Table On/Stage 2 - Set gimbals to initial attitude  ==
  Convert To Inertial : custom_blocks/Convert To Inertial
  Gimbal Input : custom_blocks/Gimbal Input
  Scope1 : Scope  NumInputPorts=3
  Toggle Attitude Reached : custom_blocks/Toggle Attitude Reached
  Zero : Constant  Value=rad2deg(HIL_Data.FDM.euler(1))  OutDataTypeStr=Inherit: Inherit via back propagation
  Zero1 : Constant  Value=rad2deg(HIL_Data.FDM.euler(2))  OutDataTypeStr=Inherit: Inherit via back propagation
  Zero2 : Constant  Value=rad2deg(HIL_Data.FDM.euler(3))  OutDataTypeStr=Inherit: Inherit via back propagation
  tag scope: Voltage2=global, stage2complete=global
  wires:
  Zero2/1 -> Scope1/3, Toggle Attitude Reached/3, Gimbal Input/3
  Zero1/1 -> Scope1/2, Toggle Attitude Reached/2, Gimbal Input/2
  Zero/1 -> Toggle Attitude Reached/1, Scope1/1, Gimbal Input/1
  Gimbal Input/1 -> [Voltage2]
  Toggle Attitude Reached/1 -> [stage2complete]
  Convert To Inertial/1 -> Gimbal Input/4, Toggle Attitude Reached/4
  [GimbalRawOutput] -> Convert To Inertial/1
  [offsets] -> Convert To Inertial/2

== system Mainframe/Flight Table/Flight Table On/Stage 3 - Track Attitude Commands ==
  Attitude Cmd : Inport
  Bus Selector1 : BusSelector  OutputSignals=Psi_rad,Theta_rad,Phi_rad
  Convert To Inertial : custom_blocks/Convert To Inertial
  Gimbal Input1 : custom_blocks/Gimbal Input
  Radians to Degrees : simulink_extras/Transformations/Radians to Degrees
  Radians to Degrees1 : simulink_extras/Transformations/Radians to Degrees
  Radians to Degrees2 : simulink_extras/Transformations/Radians to Degrees
  tag scope: Voltage3=global
  wires:
  Radians to Degrees/1 -> Gimbal Input1/1
  Radians to Degrees1/1 -> Gimbal Input1/2
  Radians to Degrees2/1 -> Gimbal Input1/3
  Bus Selector1/3 -> Radians to Degrees2/1  "<Phi_rad>"
  Bus Selector1/1 -> Radians to Degrees/1  "<Psi_rad>"
  Bus Selector1/2 -> Radians to Degrees1/1  "<Theta_rad>"
  Attitude Cmd/1 -> Bus Selector1/1
  Gimbal Input1/1 -> [Voltage3]
  Convert To Inertial/1 -> Gimbal Input1/4
  [offsets] -> Convert To Inertial/2
  [GimbalRawOutput] -> Convert To Inertial/1

== system Mainframe/Non-linear Flight Dynamic Model/Environment/Enabled Subsystem1 ==
  Enable : EnablePort
  Digital Clock : DigitalClock  SampleTime=-1
  CalibrationTime : Outport  InitialOutput=0
  wires:
  Digital Clock/1 -> CalibrationTime/1

== system Mainframe/Non-linear Flight Dynamic Model/Environment/atm_dynamic ==
  Add : Sum
  Add1 : Sum
  Bus Creator : BusCreator  Inputs=1
  Constant1 : Constant  Value=0
  Vector Concatenate : Concatenate  NumInputs=3
  course_angle_uncertainty : Constant  Value=0
  course_angle_wind : Constant  Value=0
  trafo_around_z_axis : Subsystem  mask(Transformation um z-Achse){}
      mask help: Dieser Block transformiert einen Vektor vec1 durch eine Drehung des Referenzkoordinatensystems um die z-Achse und um den Winkel gamma (in rad) in den Vektor vec2
      mask Help:
      | Name:
      | 
      |    trafo_around_z_axis
      | 
      | Beschreibung:
      | 
      |    Dieser Block transformiert einen Vektor vec1 durch eine Drehung des
      |    Referenzkoordinatensystems um die z-Achse und um den Winkel gamma
      |    (in rad) in den Vektor vec2
      | 
      | Inputs   [dimension]  [data type] [unit]:
      | 
      |     vec1    [3] [double] [-]
      |     gamma   [1] [double] [rad]
      | 
      | Outputs  [dimension]  [data type] [unit]:
      | 
      |     vec2  [3] [double] [-]
  vWW : Constant  Value=0
  vWW_uncertainty : Constant  Value=0
  vWEG : Outport  VectorParamsAs1DForOutWhenUnconnected=off
  wires:
  Bus Creator/1 -> vWEG/1  "atm_dyn_bus"
  trafo_around_z_axis/1(vec2) -> Bus Creator/1  "vWEG"
  Add1/1 -> Vector Concatenate/1
  course_angle_uncertainty/1 -> Add/2
  Constant1/1 -> Vector Concatenate/2, Vector Concatenate/3
  vWW/1 -> Add1/2
  Vector Concatenate/1 -> trafo_around_z_axis/1(vec1)
  Add/1 -> trafo_around_z_axis/2(gamma)
  vWW_uncertainty/1 -> Add1/1
  course_angle_wind/1 -> Add/1
